simulink subsystem "Thruster_Dynamics"  (R2019b)
settings: Solver=VariableStepAuto  StartTime=0.0  StopTime=10.0  RelTol=1e-3
undefined symbols (not defined in the file): T, T_inv, thrustLowerLimit, thrustUpperLimit
settings Model: Creator=esben  LastModifiedBy=esben
settings DebuggingCC: SFMachineParentedDataDiag=error

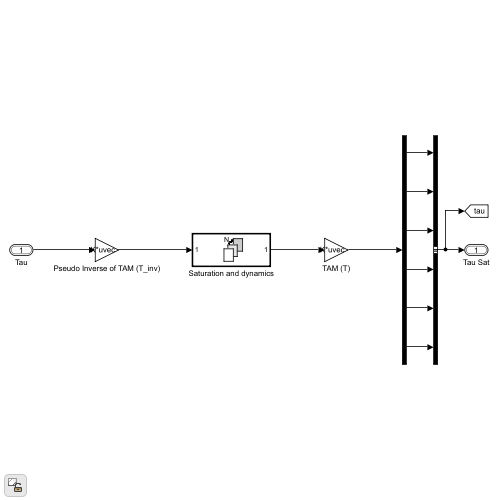
[thumbnail: Simulink's stored preview of the top-level diagram]
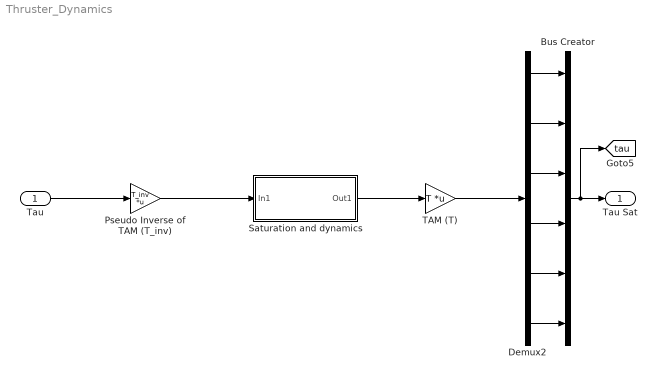
== system Thruster_Dynamics ==
  Tau : Inport  OutDataTypeStr=Bus: tau
  Bus Creator : BusCreator  Inputs=6  OutDataTypeStr=Bus: tau
      settings: InheritFromInputs=off
  Demux2 : Demux  Outputs=6
  Pseudo Inverse of TAM (T_inv) : Gain  Gain=T_inv  Multiplication=Matrix(K*u) (u vector)
  Saturation and dynamics : Subsystem  TreatAsAtomicUnit=on
  TAM (T) : Gain  Gain=T  Multiplication=Matrix(K*u) (u vector)
  Tau Sat : Outport  OutDataTypeStr=Bus: tau
  tag scope: tau=global
  wires:
  Bus Creator/1 -> Tau Sat/1, [tau]
  Tau/1 -> Pseudo Inverse of TAM (T_inv)/1
  TAM (T)/1 -> Demux2/1
  Demux2/6 -> Bus Creator/6
  Demux2/5 -> Bus Creator/5
  Demux2/4 -> Bus Creator/4
  Demux2/3 -> Bus Creator/3
  Demux2/2 -> Bus Creator/2
  Demux2/1 -> Bus Creator/1
  Pseudo Inverse of TAM (T_inv)/1 -> Saturation and dynamics/1(In1)
  Saturation and dynamics/1(Out1) -> TAM (T)/1

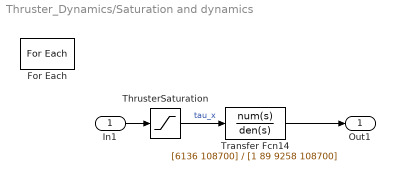
== system Thruster_Dynamics/Saturation and dynamics ==
  In1 : Inport  Partition=on  PartitionDimension=1  PartitionWidth=1  PartitionOffset=0
  For Each : ForEach  DisableCoverage=on
  ThrusterSaturation : Saturate  UpperLimit=thrustUpperLimit  LowerLimit=thrustLowerLimit  ZeroCross=off
  Transfer Fcn14 : TransferFcn  Numerator=[6136 108700]  Denominator=[1 89 9258 108700]
  Out1 : Outport  ConcatenationDimension=1
  wires:
  ThrusterSaturation/1 -> Transfer Fcn14/1  "tau_x"
  In1/1 -> ThrusterSaturation/1
  Transfer Fcn14/1 -> Out1/1
